simulink model "sensor_dump"  (R2022b)
settings: Solver=FixedStepDiscrete  StartTime=0.0  StopTime=200  FixedStep=1/30  RelTol=1e-3  EnableMultiTasking=on
values from neighbouring files (symbols this model uses):
  A = [1.06559801427  0.0478097134081  -0.0142426631232; 0.0478097134081  0.959164863261  -0.0359507847494; -0.0142426631232  -0.0359507847494  0.982079248423]    [dump1.mat]
  b = [2.14306210308 15.720848335 -0.863601368467]    [dump1.mat]
undefined symbols (not defined in the file or in its folder): Green, led0, ODR
libraries: raspberrypiIMUsensorslib x2, raspberrypiBasiclib x1
settings Model: Creator=sjohnson  LastModifiedBy=sjohnson
settings SolverCC: PositivePriorityOrder=on
settings OptimizationCC: EnhancedBackFolding=on  PassReuseOutputArgsAs=Individual arguments  ZeroExternalMemoryAtStartup=off  ZeroInternalMemoryAtStartup=off  MaxStackSize=64  OptimizeBlockOrder=speed  DifferentSizesBufferReuse=on  OptimizationCustomize=off  EfficientTunableParamExpr=on
settings DebuggingCC: ParameterTunabilityLossMsg=error
settings HardwareCC: ProdBitPerPointer=32  ProdBitPerSizeT=32  ProdBitPerPtrDiffT=32  ProdLargestAtomicInteger=Long  ProdLargestAtomicFloat=Double  ProdWordSize=32  ProdLongLongMode=on  ProdHWDeviceType=ARM Compatible->ARM Cortex  UseEmbeddedCoderFeatures=off  UseSimulinkCoderFeatures=off
settings RTWCC: Description=Embedded Coder  SystemTargetFile=ert.tlc  HardwareBoard=Raspberry Pi  TLCOptions="-aInlineSetEventsForThisBaseRateFcn=TLC_FALSE -aSuppressMultiTaskScheduler=TLC_FALSE  -aRateBasedStepFcn=0"  TemplateMakefile=ert_default_tmf  Toolchain=GNU GCC Embedded Linux  BuildConfiguration=Faster Runs
settings CodeAppCC: ForceParamTrailComments=on  IgnoreCustomStorageClasses=off  OperatorAnnotations=on  SimulinkDataObjDesc=on  SFDataObjDesc=on  InsertBlockDesc=on
settings ERTTargetCC: SupportNonInlinedSFcns=on  SupportVariableSizeSignals=on  ExtModeTransport=2  ExtModeStaticAlloc=on  ExtModeMexFile=ext_xcp  ExtModeIntrfLevel=Level2 - Open

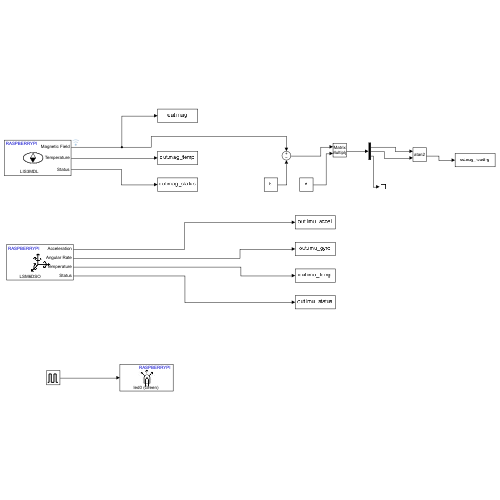
[thumbnail: Simulink's stored preview of the top-level diagram]
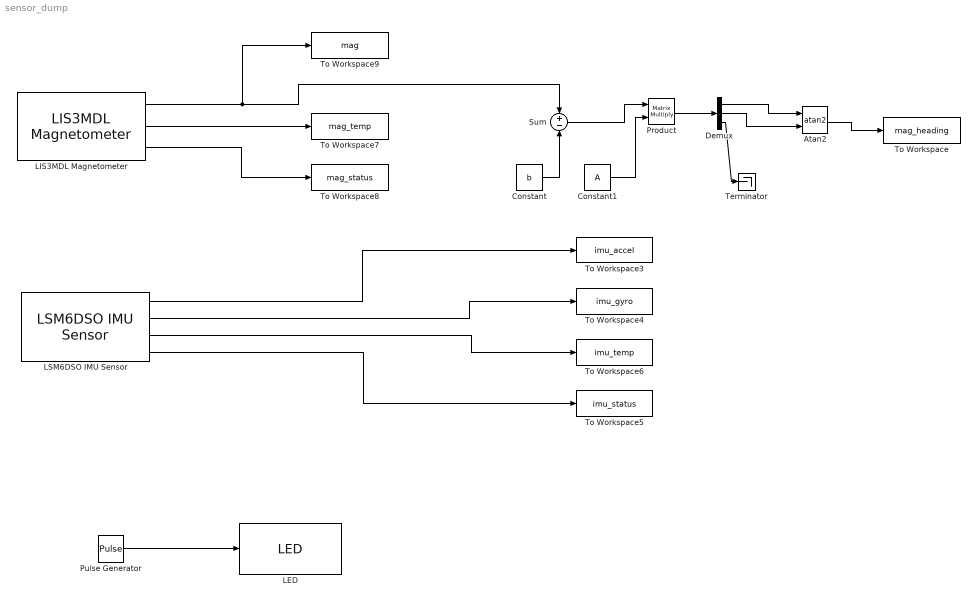
== system sensor_dump ==
  Atan2 : Trigonometry  Operator=atan2
  Constant : Constant  Value=b
  Constant1 : Constant  Value=A
  Demux : Demux  Outputs=3
  LED : raspberrypiBasiclib/LED  BoardProperty=Pi 4 Model B  LED_=led0 (Green)
  LIS3MDL Magnetometer : raspberrypiIMUsensorslib/LIS3MDL Magnetometer  I2CModule=1  I2CAddress=0x1E  IsActiveMagnetometer=on  IsActiveTemperature=on  IsStatus=on  SampleTime=-1  MagnetometerRange=+/- 400 uT  MagnetometerODR=40 Hz
  LSM6DSO IMU Sensor : raspberrypiIMUsensorslib/LSM6DSO IMU Sensor  I2CModule=1  I2CAddress=0x6B  IsActiveAcceleration=on  IsActiveAngularRate=on  IsActiveTemperature=on  IsActiveStatus=on  IsActiveTimeStamp=off  SampleTime=-1  QueueSizeFactor=3  AccelerometerRange=+/- 2g  AccelerometerODR=52 Hz  AccelSelectCompositeFilter=No filter  AccelLPF2BW=ODR/4  AccelHPFBW=ODR/4  GyroscopeRange=1000 dps  GyroscopeODR=52 Hz  EnableGyroHPF=off  GyroHPFBW=0.016 Hz  EnableGyroLPF=off  GyroLPFBWMode=0
  Product : Product  Multiplication=Matrix(*)
  Pulse Generator : DiscretePulseGenerator  PulseType=Time based  Period=20  PulseWidth=25
  Sum : Sum  Inputs=+-
  Terminator : Terminator
  To Workspace : ToWorkspace  VariableName=mag_heading  SaveFormat=Structure With Time  SampleTime=-1
  To Workspace3 : ToWorkspace  VariableName=imu_accel  SaveFormat=Structure With Time  SampleTime=-1
  To Workspace4 : ToWorkspace  VariableName=imu_gyro  SaveFormat=Structure With Time  SampleTime=-1
  To Workspace5 : ToWorkspace  VariableName=imu_status  SaveFormat=Structure With Time  SampleTime=-1
  To Workspace6 : ToWorkspace  VariableName=imu_temp  SaveFormat=Structure With Time  SampleTime=-1
  To Workspace7 : ToWorkspace  VariableName=mag_temp  SaveFormat=Structure With Time  SampleTime=-1
  To Workspace8 : ToWorkspace  VariableName=mag_status  SaveFormat=Structure With Time  SampleTime=-1
  To Workspace9 : ToWorkspace  VariableName=mag  SaveFormat=Structure With Time  SampleTime=-1
  wires:
  LIS3MDL Magnetometer/1 -> To Workspace9/1, Sum/1
  Sum/1 -> Product/1
  Constant1/1 -> Product/2
  LSM6DSO IMU Sensor/4 -> To Workspace5/1
  LIS3MDL Magnetometer/3 -> To Workspace8/1
  LSM6DSO IMU Sensor/2 -> To Workspace4/1
  Demux/3 -> Terminator/1
  LIS3MDL Magnetometer/2 -> To Workspace7/1
  LSM6DSO IMU Sensor/1 -> To Workspace3/1
  Product/1 -> Demux/1
  LSM6DSO IMU Sensor/3 -> To Workspace6/1
  Constant/1 -> Sum/2
  Demux/1 -> Atan2/1
  Demux/2 -> Atan2/2
  Atan2/1 -> To Workspace/1
  Pulse Generator/1 -> LED/1
